simulink model "TPGex"  (Simulink 8.5)
settings: Solver=FixedStepDiscrete  SolverMode=SingleTasking  StartTime=0.0  StopTime=0.1  FixedStep=1e-4  RelTol=1e-3  AbsTol=1e-6
libraries: inputs x1
settings Model: Creator=PC  LastModifiedBy=PC
settings DataIOCC: LimitDataPoints=off
settings OptimizationCC: BlockReduction=off  BooleanDataType=off  ExpressionDepthLimit=128
settings DebuggingCC: SaveWithParameterizedLinksMsg=none  SignalResolutionControl=TryResolveAllWithWarning  MultiTaskDSMMsg=warning  MultiTaskCondExecSysMsg=none  FcnCallInpInsideContextMsg=EnableAllAsError  StateNameClashWarn=none  StrictBusMsg=None
settings HardwareCC: TargetUnknown=on

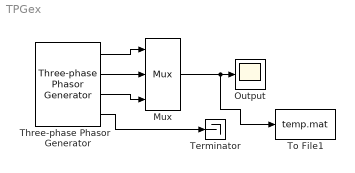
== system TPGex ==
  Mux : Mux  Inputs=3
  Output : Scope
      settings: TickLabels=on  YMin=-10  YMax=10
  Terminator : Terminator
  Three-phase Phasor   Generator : inputs/Three-phase Phasor   Generator  phase_type=Phase quantities-unsymmetrical  phase1=[5 45]  phase2=[2 0]  phase3=[1 -30]  f=60  to=1/60
  To File1 : ToFile  Filename=temp.mat  MatrixName=sig
  wires:
  Three-phase Phasor   Generator/1 -> Mux/1
  Three-phase Phasor   Generator/2 -> Mux/2
  Three-phase Phasor   Generator/3 -> Mux/3
  Three-phase Phasor   Generator/4 -> Terminator/1
  Mux/1 -> To File1/1, Output/1
